simulink model "simpledemo01"  (Simulink 7.6)
settings: Solver=FixedStepDiscrete  StartTime=0.0  StopTime=10.0  FixedStep=Auto  RelTol=1e-3
PreLoadFcn:
  | ParamA=1;
  | ParamB=2;
undefined symbols (not defined in the file or in its folder): sldvsubsys
libraries: sldvlib x3, simulink x1
settings Model: Creator=itoy  LastModifiedBy=itoy
settings DataIOCC: LimitDataPoints=off  SaveFormat=StructureWithTime  SaveOutput=off  SaveTime=off
settings OptimizationCC: OptimizeModelRefInitCode=on  LifeSpan=1
settings DebuggingCC: FcnCallInpInsideContextMsg=Enable All  StrictBusMsg=Warning
settings RTWCC: SystemTargetFile=ert.tlc  GenCodeOnly=on  TemplateMakefile=ert_default_tmf  Description=Real-Time Workshop Embedded Coder  GenerateReport=on  ProcessScript=ert_make_rtw_hook  IncludeHyperlinkInReport=on  LaunchReport=on  GenerateTraceInfo=on  GenerateTraceReport=on  GenerateTraceReportSl=on  GenerateTraceReportSf=on  GenerateTraceReportEml=on
settings CodeAppCC: IgnoreCustomStorageClasses=off
settings ERTTargetCC: MultiwordLength=2048  GenerateSampleERTMain=on  ERTCustomFileTemplate=example_file_process.tlc  ConvertIfToSwitch=off

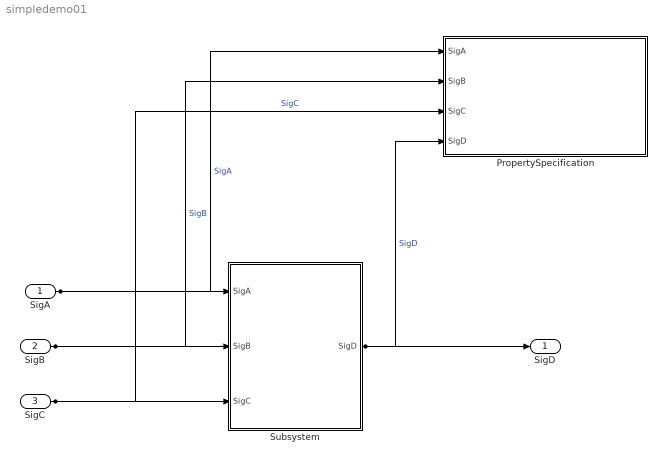
== system simpledemo01 ==
  SigA : Inport
  SigB : Inport  Port=2
  SigC : Inport  Port=3
  PropertySpecification : Subsystem  Tag=VerificationSubsystem  DisableCoverage=on  LoadFcn=sldvsubsys('check')  TreatAsAtomicUnit=on  SimViewingDevice=on  mask(VerificationSubsystem){}
      mask help: aa
      mask init:
      | sldvsubsys('maskInit');
      settings: OpenFcn=PropertySpecificationUI('Block',gcb)
      settings: CopyFcn=|
      | sldvsubsys('copy');
      |  set_param(gcb,'LinkStatus','none')
      settings: PreSaveFcn=|
      | set_param(gcb,'SimViewingDevice','on');
      | sldvsubsys('check');
      mask Help: helpview(fullfile(docroot,'toolbox','sldv','sldv.map'),'verificationsubsystem')
      mask Display: image(imread('sldvicon_versubsys.png','BackGroundColor',[1 1 1]),'center');
  Subsystem : Subsystem
  SigD : Outport
  wires:
  SigA/1 -> Subsystem/1(SigA), PropertySpecification/1(SigA)  "SigA"
  SigB/1 -> Subsystem/2(SigB), PropertySpecification/2(SigB)  "SigB"
  SigC/1 -> Subsystem/3(SigC), PropertySpecification/3(SigC)  "SigC"
  Subsystem/1(SigD) -> SigD/1, PropertySpecification/4(SigD)  "SigD"

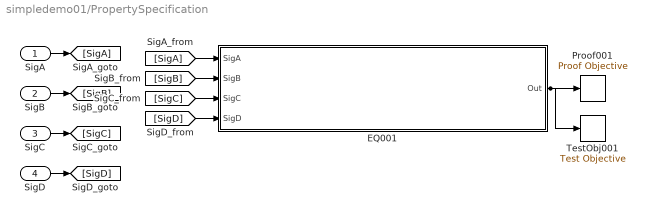
== system simpledemo01/PropertySpecification ==
  SigA : Inport
  SigB : Inport  Port=2
  SigC : Inport  Port=3
  SigD : Inport  Port=4
  EQ001 : Subsystem  Tag=CustomScope  mask(sldvLiteralTemporalLogicLib){InputVar=SigA,SigB,SigC,SigD, ParamVar=ParamA,ParamB, VerifEq=SigA > 0 && ( SigB + SigC < ParamA) ==> SigD == ParamB}
      mask prompts: InputVar "入力変数"; ParamVar "パラメータ変数"; VerifEq "検査式"
      mask help: sldvLiteralTemporalLogiclib
      mask init:
      | literalEq2SimulinkCallback(gcb,InputVar,ParamVar,VerifEq)
      mask Display: disp(VerifEq)
  Proof001 : sldvlib/Proof Objective  SystemSampleTime=-1  enabled=on  customAVTBlockType=Proof Objective  intervals=true  dispValues=on  outEnabled=off  enableStopSim=off
      settings: AttributesFormatString=%<intervals>
  TestObj001 : sldvlib/Test Objective  SystemSampleTime=-1  enabled=off  customAVTBlockType=Test Objective  intervals=true  dispValues=on  outEnabled=off
      settings: AttributesFormatString=%<intervals>
  wires:
  SigA/1 -> [SigA]
  SigB/1 -> [SigB]
  SigC/1 -> [SigC]
  SigD/1 -> [SigD]
  [SigA] -> EQ001/1(SigA)
  [SigB] -> EQ001/2(SigB)
  [SigC] -> EQ001/3(SigC)
  [SigD] -> EQ001/4(SigD)
  EQ001/1(Out) -> Proof001/1, TestObj001/1

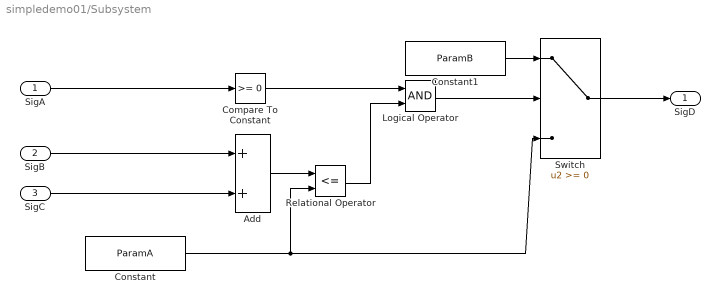
== system simpledemo01/Subsystem ==
  SigA : Inport
  SigB : Inport  Port=2
  SigC : Inport  Port=3
  Add : Sum
  Compare To Constant : simulink/Logic and Bit Operations/Compare To Constant  SystemSampleTime=-1  relop=>=  const=0  LogicOutDataTypeMode=uint8
  Constant : Constant  Value=ParamA
  Constant1 : Constant  Value=ParamB
  Logical Operator : Logic  AllPortsSameDT=off  OutDataTypeStr=boolean
  Relational Operator : RelationalOperator  Operator=<=  OutDataTypeStr=boolean
  Switch : Switch
  SigD : Outport
  wires:
  SigB/1 -> Add/1
  SigC/1 -> Add/2
  SigA/1 -> Compare To Constant/1
  Compare To Constant/1 -> Logical Operator/1
  Add/1 -> Relational Operator/1
  Constant/1 -> Relational Operator/2, Switch/3
  Relational Operator/1 -> Logical Operator/2
  Logical Operator/1 -> Switch/2
  Constant1/1 -> Switch/1
  Switch/1 -> SigD/1

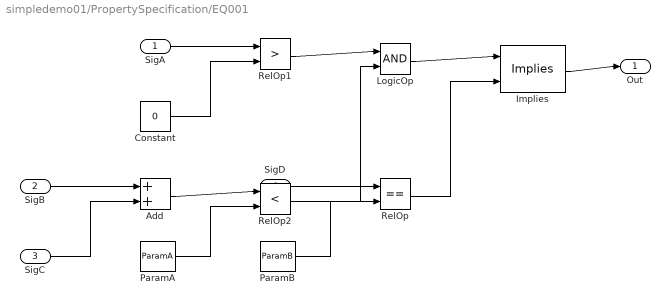
== system simpledemo01/PropertySpecification/EQ001 ==
  SigA : Inport
  SigB : Inport  Port=2
  SigC : Inport  Port=3
  SigD : Inport  Port=4
  Add : Sum
  Constant : Constant  Value=0  OutDataTypeStr=Inherit: Inherit via back propagation
  Implies : sldvlib/Implies  SystemSampleTime=-1
  LogicOp : Logic  AllPortsSameDT=off  OutDataTypeStr=boolean
  ParamA : Constant  Value=ParamA
  ParamB : Constant  Value=ParamB
  RelOp : RelationalOperator  Operator===  OutDataTypeStr=boolean
  RelOp1 : RelationalOperator  Operator=>  OutDataTypeStr=boolean
  RelOp2 : RelationalOperator  Operator=<  OutDataTypeStr=boolean
  Out : Outport
  wires:
  Implies/1 -> Out/1
  SigB/1 -> Add/1
  LogicOp/1 -> Implies/1
  RelOp1/1 -> LogicOp/1
  SigD/1 -> RelOp/1
  SigA/1 -> RelOp1/1
  Add/1 -> RelOp2/1
  ParamA/1 -> RelOp2/2
  ParamB/1 -> RelOp/2
  SigC/1 -> Add/2
  Constant/1 -> RelOp1/2
  RelOp/1 -> Implies/2
  RelOp2/1 -> LogicOp/2
